simulink model "PC_MSFS_STATION"  (R2021b)
settings: Solver=FixedStepAuto  StartTime=0.0  StopTime=2000  FixedStep=0.03  RelTol=1e-3
undefined symbols (not defined in the file): CONTROL, DiscIntNeverNeededParam, f, MODEL, MODEL_INI
libraries: instrumentlib x22, SimConnectToolbox x3, simulink x2
(part 2 of 2)

== matlab function PC_MSFS_STATION/SYSTEM/UNICYCLE MODEL ==
  data: STATE input; STATE_DERIVATIVE output; MODEL_IN input; MODEL output Bus: MODEL_Bus
function [STATE_DERIVATIVE,MODEL] = SO_UNICYCLE_MODEL(STATE, MODEL_IN)
% COPY MODEL BUS
MODEL = MODEL_IN;
%--------------------------------------------------------------------------
% SO UNICYCLE PARAMETERS
%--------------------------------------------------------------------------
dist_p = MODEL.PARAM.DISP_P;
at_wp = MODEL.INPUT.AT_WP;
%--------------------------------------------------------------------------
% SIMULATION PARAMETERS
%--------------------------------------------------------------------------
flight_status = MODEL.PARAM.FLIGHT_STATUS;
heading_offset = MODEL.PARAM.HEADING_OFFSET;
%--------------------------------------------------------------------------
% SAVE OLD GEOMETRIC COORDINATES
%--------------------------------------------------------------------------
prev_lat = MODEL.OUTPUT.LATITUDE;
prev_long = MODEL.OUTPUT.LONGITUDE;
prev_head = MODEL.OUTPUT.HEADING;
prev_head_NED = MODEL.OUTPUT.HEADING_NED;
%--------------------------------------------------------------------------
% EVALUATE FLIGHT STATUS
%--------------------------------------------------------------------------
if flight_status < 1 % Only reading values from MSFS
    % INITIALIZATION
    theta_long = MODEL.INPUT.LONGITUDE;
    phi_lat = MODEL.INPUT.LATITUDE;
    % altitude = MODEL.INPUT.ALTITUDE;
    altitude = MODEL.OUTPUT.ALTITUDE;
    rho = altitude + 20.902e6;
    % Displaced Point Dynamics Y = {y1, y2, vy1, vy2}
    y1 = rho*cos(phi_lat)*cos(theta_long);
    y2 = rho*cos(phi_lat)*sin(theta_long);
    vy1 = 0;
    vy2 = 0;
    % Center of Mass Dynamics X = {x1, x2, s, theta, omega}
    s = 0;
    theta = 0;
    omega = 0;
    x1 = y1 - dist_p*cos(theta);
    x2 = y2 - dist_p*sin(theta);
else % Reading and writing on MSFS
    %--------------------------------------------------------------------------
    % UPDATE STATE VARIABLES
    %--------------------------------------------------------------------------
    % Displaced Point Dynamics Y = {y1, y2, vy1, vy2}
    y1 = STATE(1);
    y2 = STATE(2);
    vy1 = STATE(3);
    vy2 = STATE(4);
    % Center of Mass Dynamics X = {x1, x2, s, theta, omega}
    s = STATE(5);
    theta = STATE(6);
    omega = STATE(7);
    x1 = y1 - dist_p*cos(theta);
    x2 = y2 - dist_p*sin(theta);
    % Update Latitude and Longitude
    altitude = MODEL.OUTPUT.ALTITUDE;
    rho = altitude + 20.902e6;
    if y1 >=0
        % First or fourth quadrant
        if y2 >=0
            %First quadrant
            theta_long = atan(abs(y2)/abs(y1));
        else
            % Fourth quadrant
            %         theta_long = 2*pi - atan(abs(y2)/abs(y1));
            theta_long = - atan(abs(y2)/abs(y1));
        end
    else
        % Second or third quadrant
        if y2 >=0
            % Second quadrant
            theta_long = pi - atan(abs(y2)/abs(y1));
        else
            % Third quadrant
            theta_long = pi + atan(abs(y2)/abs(y1));
        end
    end
    phi_lat = acos(y1/(rho*cos(theta_long)));
end
%--------------------------------------------------------------------------
% HEADING CONTROL
%--------------------------------------------------------------------------
% CHANGE OF FRAME FROM XYZ TO NED
sinPOS_Lat = sin(phi_lat);
cosPOS_Lat = cos(phi_lat);
sinPOS_Long = sin(theta_long);
cosPOS_Long = cos(theta_long);

Iner_to_NED = zeros(3,3);
Iner_to_NED(1,1) = - sinPOS_Lat*cosPOS_Long;
Iner_to_NED(2,1) = - sinPOS_Long;
Iner_to_NED(3,1) = - cosPOS_Lat*cosPOS_Long;
Iner_to_NED(1,2) = - sinPOS_Lat*sinPOS_Long;
Iner_to_NED(2,2) = cosPOS_Long;
Iner_to_NED(3,2) = - cosPOS_Lat*sinPOS_Long;
Iner_to_NED(1,3) = cosPOS_Lat;
Iner_to_NED(2,3) = 0;
Iner_to_NED(3,3) = - sinPOS_Lat;

NED_vy = Iner_to_NED*[vy1;vy2;0];
NED_vy1 = NED_vy(1); % NORTH
NED_vy2 = NED_vy(2); % EAST
heading_NED = atan2(NED_vy2,NED_vy1) + heading_offset;
heading = atan2(vy2,vy1) + heading_offset;
%--------------------------------------------------------------------------
% INPUTS
%--------------------------------------------------------------------------
tau1 = MODEL.INPUT.TAU1;
tau2 = MODEL.INPUT.TAU2;
%--------------------------------------------------------------------------
% STATE EQUATIONS
%--------------------------------------------------------------------------
y1dot = vy1;
y2dot = vy2;
y1ddot = tau1;
y2ddot = tau2;
sdot = -omega^2*dist_p + tau1*cos(theta) + tau2*sin(theta);
thetadot = omega;
omegadot = 1/dist_p*(omega*s - tau1*sin(theta) + tau2*cos(theta));
%--------------------------------------------------------------------------
% STATE DERIVATIVES
%--------------------------------------------------------------------------
STATE_DERIVATIVE = [y1dot; y2dot; y1ddot; y2ddot; sdot; thetadot; omegadot];
%%%%%%%%%%%%%%%%%%%%%%%%%%%%%%%%%%%%%%%%%%%%%%%%%%%%%%%%%%%%%%%%%%%%%%%%%%%
% OUTPUT BUS
%%%%%%%%%%%%%%%%%%%%%%%%%%%%%%%%%%%%%%%%%%%%%%%%%%%%%%%%%%%%%%%%%%%%%%%%%%%
MODEL.STATE = [y1 ; y2 ; vy1 ; vy2 ; s ; theta ; omega];
MODEL.OUTPUT.X1 = x1;
MODEL.OUTPUT.X2 = x2;
MODEL.OUTPUT.X = sqrt(x1^2 + x2^2);
MODEL.OUTPUT.Y = sqrt(y1^2 + y2^2);

MODEL.OUTPUT.LATITUDE = phi_lat;
MODEL.OUTPUT.LONGITUDE = theta_long;
MODEL.OUTPUT.HEADING = heading;
MODEL.OUTPUT.HEADING_NED = heading_NED;
% if at_wp == 0
%     MODEL.OUTPUT.LATITUDE = phi_lat;
%     MODEL.OUTPUT.LONGITUDE = theta_long;
%     MODEL.OUTPUT.HEADING = heading;
%     MODEL.OUTPUT.HEADING_NED = heading_NED;
% else
%     MODEL.OUTPUT.LATITUDE = prev_lat;
%     MODEL.OUTPUT.LONGITUDE = prev_long;
%     MODEL.OUTPUT.HEADING = prev_head;
%     MODEL.OUTPUT.HEADING_NED = prev_head_NED;
% end
return
